simulink model "HVDC_VSC_1CPUcore_dcpl"  (Simulink 8.4)
settings: Solver=ode3  SolverMode=SingleTasking  StartTime=0.0  StopTime=70.0  FixedStep=Ts_Power  RelTol=1e-3  AbsTol=1e-2
PreLoadFcn:
  | Ts_Power=50e-6; Ts_Control=1*Ts_Power; init_cosim_IA; startup_transients_hvdc_vsc;
PostLoadFcn:
  | Ts_Power=50e-6; Ts_Control=1*Ts_Power; init_cosim_IA; startup_transients_hvdc_vsc;
InitFcn:
  | Ts_Power=50e-6; Ts_Control=1*Ts_Power; init_cosim_IA; startup_transients_hvdc_vsc;
values from neighbouring files (symbols this model uses):
  h = 5    [init_cosim_IA.m]
  intfDelay = 400.0    (= 400)    [init_cosim_IA.m]
  Ts_intf = 2*Ts_Power    [init_cosim_IA.m]
undefined symbols (not defined in the file or in its folder): CLARK, D1, Delta, dPref1_2, dPref1_2_rlimit, gcbh, level, lib_mesures, magnitude, ResistanceM, rte_drive_private_lib, rte_tsb3level_hiz_rect_cb, sps_rtmsupport, t_deblock_Pref1, t_deblock_Udref2, t_dPref1_2, t_init_AC, t_SwitchITMIdc, t_SwitchITMVdc, t_vsag_end, t_vsag_start, TSB3_hiZR
libraries: powerlib x162, powerlib_extras x71, spsVIMeasurementModel x63, rteventslib x26, op_dpl_lib x14, powerlib_meascontrol x14, rtlab x6, sps_avr x3, artemis x1
(part 1 of 11)
Description:
  | The 'Model  initialization function' defined in the
  | 
  | Model Properties automatically sets the sample time
  | 
  | Ts to 50e-6 s
settings Model: ARTEMISmethode_block_infos=$$__separator__$$HVDC_VSC_1CPUcore_dcpl/ARTEMIS Guide$$__separator__$$  Creator=Gilbert Sybille, IREQ  LastModifiedBy=maja  CovSFcnEnable=on  ExtModeTrigMode=oneshot  ExtModeArmWhenConnect=off  ExtModeAutoUpdateStatusClock=off  BufferReuse=off
settings DataIOCC: LimitDataPoints=off  SaveFormat=StructureWithTime  SaveOutput=off  DSMLogging=off  SaveTime=off  SignalLoggingName=sigsOut
settings OptimizationCC: BlockReduction=off  BooleanDataType=off  OptimizeBlockIOStorage=off  BufferReuse=off  GlobalBufferReuse=off  ExpressionFolding=off  LocalBlockOutputs=off  InitFltsAndDblsToZero=on
settings DebuggingCC: SaveWithParameterizedLinksMsg=none  CheckExecutionContextPreStartOutputMsg=on  CheckExecutionContextRuntimeOutputMsg=on  SignalResolutionControl=TryResolveAllWithWarning  SolverPrmCheckMsg=none  MultiTaskDSMMsg=warning  MultiTaskCondExecSysMsg=none  FcnCallInpInsideContextMsg=EnableAllAsWarning  UnconnectedInputMsg=none  UnconnectedOutputMsg=none  UnconnectedLineMsg=none  FrameProcessingCompatibilityMsg=error
settings HardwareCC: TargetHWDeviceType=32-bit Generic  ProdEqTarget=off
settings GRTTargetCC: TargetFcnLib=ansi_tfl_tmw.mat

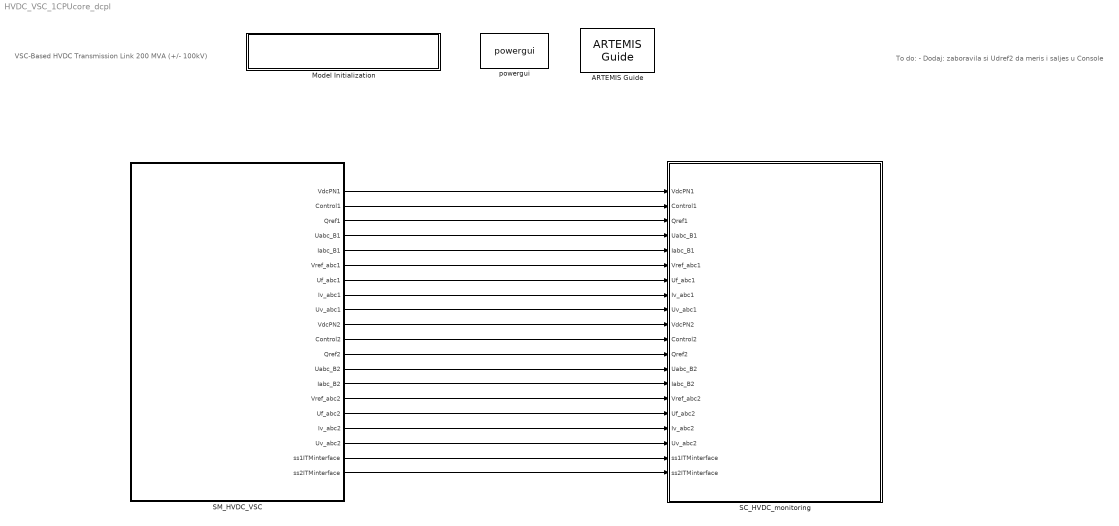
== system HVDC_VSC_1CPUcore_dcpl ==
  note: VSC-Based HVDC Transmission Link
      | 200 MVA  (+/- 100kV)
  note: To do:
      | - Dodaj: zaboravila si Udref2 da meris i saljes u Console
  ARTEMIS Guide : artemis/ARTEMIS/ARTEMIS Guide  Tag=FTSSmethode_opal_4hx0r99  Description=5.0_z1  lock=on  Ts=Ts_Power  opt=art5  dyna=off  nb_perm=4  RT_fullcomp=off  ssn=off  ssn_itvc=off  ssn_ivic=off  ssn_ext=off  ssn_solver=Trapezoidal  ssn_impulse=off  ssn_quasimpulse=off  ssn_impulse_loop=5  paraExtinctionThy=off  Thy_Impulse=on  dtc=Off  dtc_opt=normal  ao=on  simtype=off  ct_mac=off  lin_mov=off  lsp=[0.001 2]  spike_skip=Disabled  dtc_extra=1  dtc_sws=normal  dtc_pied=0.5  SPSRulesBlock=SPSRules  tre=on  ctmm=off  LF=off  dpl_type=ARTEMiS DPL  rlc_type=off  custom_type=off  para=on  ssn_ImpulseLoopBlockedStateUpdate=5  ssn_mov_iter_number=5  ssn_switch_iter_number=5
  Model Initialization : Subsystem  mask(Model Functions){InitFcnX=Ts_Power=50e-6; Ts_Control=1*Ts_Power; init_cosim_IA; startup_transients_hvdc_vsc;, prel=on, posl=on, inif=on, strf=off}
      mask prompts: InitFcnX "Initialisation"; prel "Preload Function"; posl "PostLoad Function"; inif "InitFcn"; strf "StartFcn"
      mask init:
      | currentBlock = gcb;
      | root = bdroot(currentBlock);
      | 
      | if ~strcmp(get_param(root,'BlockDiagramType'),'library')
      |     if prel==1
      |         set_param(root, 'PreLoadFcn', InitFcnX);
      |     else
      |         set_param(root, 'PreLoadFcn', '');
      |     end
      |     if inif==1
      |         set_param(root, 'InitFcn', InitFcnX);
      |     else
      |         set_param(root, 'InitFcn', '');
      |     end
      |     if strf==1
      |         set_param(root, 'StartFcn', InitFcnX);
      |     else
      |         set_param(root, 'StartFcn', '');
      |     end
      |     if posl==1
      |         set_param(root, 'PostLoadFcn', InitFcnX);
      |     else
      |         set_param(root, 'PostLoadFcn', '');
      |     end
      | end
      | 
      | pos = get_param(currentBlock, 'Position');
      | width = pos(3) - pos(1); height = pos(4) - pos(2);
      | txt = [ upper(root) '\n' '- InitFcn. . . . . '  get_param(root, 'InitFcn') ];
      settings: CopyFcn=set_param(gcb,'LinkStatus','none')
      mask Display: text(5, height*0.5, txt, 'horizontalAlignment', 'left', 'verticalAlignment', 'middle') ;
  SC_HVDC_monitoring : Subsystem
  SM_HVDC_VSC : Subsystem
  powergui : powerlib/powergui  Priority=2  SimulationMode=Discrete  SolverType=Tustin  SampleTime=Ts_Power  frequency=60  SPID=off  DisableSnubberDevices=off  DisableRonSwitches=off  DisableVfSwitches=off  SwTol=0  DisplayEquations=off  Interpol=off  methode=off  Ts=0  frequencyindice=0  Pbase=100e6  ErrMax=1e-4  Iterations=50  UnitsV=kV  UnitsW=MW  FunctionMessages=off  echomessages=on  HookPort=off  EnableUseOfTLC=off  x0status=zero  RestoreLinks=warning  ResistiveCurrentMeasurement=off  Frange=[0:2:500]  Ylog=off  Xlog=on  ShowGrid=off  save=off  variable=ZData  structure=res_fft  ZoomFFT=on  StartTime=1.5  cycles=2  DisplayStyle=1  fundamental=50  FreqAxis=off  MaxFrequency=3000  frequencyindicesteady=1  RmsSteady=1  display=off
  wires:
  SM_HVDC_VSC/1(VdcPN1) -> SC_HVDC_monitoring/1(VdcPN1)
  SM_HVDC_VSC/2(Control1) -> SC_HVDC_monitoring/2(Control1)
  SM_HVDC_VSC/3(Qref1) -> SC_HVDC_monitoring/3(Qref1)
  SM_HVDC_VSC/4(Uabc_B1) -> SC_HVDC_monitoring/4(Uabc_B1)
  SM_HVDC_VSC/5(Iabc_B1) -> SC_HVDC_monitoring/5(Iabc_B1)
  SM_HVDC_VSC/6(Vref_abc1) -> SC_HVDC_monitoring/6(Vref_abc1)
  SM_HVDC_VSC/7(Uf_abc1) -> SC_HVDC_monitoring/7(Uf_abc1)
  SM_HVDC_VSC/8(Iv_abc1) -> SC_HVDC_monitoring/8(Iv_abc1)
  SM_HVDC_VSC/9(Uv_abc1) -> SC_HVDC_monitoring/9(Uv_abc1)
  SM_HVDC_VSC/10(VdcPN2) -> SC_HVDC_monitoring/10(VdcPN2)
  SM_HVDC_VSC/11(Control2) -> SC_HVDC_monitoring/11(Control2)
  SM_HVDC_VSC/12(Qref2) -> SC_HVDC_monitoring/12(Qref2)
  SM_HVDC_VSC/13(Uabc_B2) -> SC_HVDC_monitoring/13(Uabc_B2)
  SM_HVDC_VSC/14(Iabc_B2) -> SC_HVDC_monitoring/14(Iabc_B2)
  SM_HVDC_VSC/15(Vref_abc2) -> SC_HVDC_monitoring/15(Vref_abc2)
  SM_HVDC_VSC/16(Uf_abc2) -> SC_HVDC_monitoring/16(Uf_abc2)
  SM_HVDC_VSC/17(Iv_abc2) -> SC_HVDC_monitoring/17(Iv_abc2)
  SM_HVDC_VSC/18(Uv_abc2) -> SC_HVDC_monitoring/18(Uv_abc2)
  SM_HVDC_VSC/19(ss1ITMinterface) -> SC_HVDC_monitoring/19(ss1ITMinterface)
  SM_HVDC_VSC/20(ss2ITMinterface) -> SC_HVDC_monitoring/20(ss2ITMinterface)

== system HVDC_VSC_1CPUcore_dcpl/Model Initialization ==

== system HVDC_VSC_1CPUcore_dcpl/SC_HVDC_monitoring ==
  VdcPN1 : Inport
  Control1 : Inport  Port=2
  Qref1 : Inport  Port=3
  Uabc_B1 : Inport  Port=4
  Iabc_B1 : Inport  Port=5
  Vref_abc1 : Inport  Port=6
  Uf_abc1 : Inport  Port=7
  Iv_abc1 : Inport  Port=8
  Uv_abc1 : Inport  Port=9
  VdcPN2 : Inport  Port=10
  Control2 : Inport  Port=11
  Qref2 : Inport  Port=12
  Uabc_B2 : Inport  Port=13
  Iabc_B2 : Inport  Port=14
  Vref_abc2 : Inport  Port=15
  Uf_abc2 : Inport  Port=16
  Iv_abc2 : Inport  Port=17
  Uv_abc2 : Inport  Port=18
  ss1ITMinterface : Inport  Port=19
  ss2ITMinterface : Inport  Port=20
  Bus Selector : BusSelector  OutputSignals=ss1VdcPOSf,ss1VdcNEGf,ss1VdcLINKf,ss1IdcPOSf,ss1IdcNEGf,ss1Pdcf
  Bus Selector1 : BusSelector  OutputSignals=ss2VdcPOSf,ss2VdcNEGf,ss2VdcLINKf,ss2IdcPOSf,ss2IdcNEGf,ss2Pdcf
  Data Acquisition Station 1 : Subsystem
      mask Display: disp('Open this block\nto visualize\nrecorded signals')
  Data Acquisition Station 2 : Subsystem
      mask Display: disp('Open this block\nto visualize\nrecorded signals')
  OpComm : rtlab/OpComm  nbport=9  groupe_acq=1  subsys_rate=Ts_Power  st=0  Synchronization=on  Interpolation=on  Threshold=1.0  Missed_Data=off  Sim_Time=off  Samples=off  dynSigOut=off  from_console=0  warning_done=off  writeOpCommFile=off  Offset=off
  OpComm1 : rtlab/OpComm  nbport=9  groupe_acq=2  subsys_rate=Ts_Power  st=0  Synchronization=on  Interpolation=on  Threshold=1.0  Missed_Data=off  Sim_Time=off  Samples=off  dynSigOut=off  from_console=0  warning_done=off  writeOpCommFile=off  Offset=off
  OpComm2 : rtlab/OpComm  nbport=1  groupe_acq=3  subsys_rate=Ts_Power  st=0  Synchronization=on  Interpolation=on  Threshold=1.0  Missed_Data=off  Sim_Time=off  Samples=off  dynSigOut=off  from_console=0  warning_done=off  writeOpCommFile=off  Offset=off
  OpComm3 : rtlab/OpComm  nbport=1  groupe_acq=4  subsys_rate=Ts_Power  st=0  Synchronization=on  Interpolation=on  Threshold=1.0  Missed_Data=off  Sim_Time=off  Samples=off  dynSigOut=off  from_console=0  warning_done=off  writeOpCommFile=off  Offset=off
  Subsystem : Subsystem
  wires:
  VdcPN1/1 -> OpComm/1
  Control1/1 -> OpComm/2
  Qref1/1 -> OpComm/3
  Uabc_B1/1 -> OpComm/4
  Iabc_B1/1 -> OpComm/5
  Vref_abc1/1 -> OpComm/6
  Uf_abc1/1 -> OpComm/7
  Iv_abc1/1 -> OpComm/8
  Uv_abc1/1 -> OpComm/9
  OpComm/1 -> Data Acquisition Station 1/1(VdcPN1)
  OpComm/2 -> Data Acquisition Station 1/2(Control1)
  OpComm/3 -> Data Acquisition Station 1/3(Qref1)
  OpComm/4 -> Data Acquisition Station 1/4(Uabc_B1)
  OpComm/5 -> Data Acquisition Station 1/5(Iabc_B1)
  OpComm/6 -> Data Acquisition Station 1/6(Vref_abc1)
  OpComm/7 -> Data Acquisition Station 1/7(Uf_abc1)
  OpComm/8 -> Data Acquisition Station 1/8(Iv_abc1)
  OpComm/9 -> Data Acquisition Station 1/9(Uv_abc1)
  VdcPN2/1 -> OpComm1/1
  Control2/1 -> OpComm1/2
  Qref2/1 -> OpComm1/3
  Uabc_B2/1 -> OpComm1/4
  Iabc_B2/1 -> OpComm1/5
  Vref_abc2/1 -> OpComm1/6
  Uf_abc2/1 -> OpComm1/7
  Iv_abc2/1 -> OpComm1/8
  Uv_abc2/1 -> OpComm1/9
  OpComm1/1 -> Data Acquisition Station 2/1(VdcPN2)
  OpComm1/2 -> Data Acquisition Station 2/2(Control2)
  OpComm1/3 -> Data Acquisition Station 2/3(Qref2)
  OpComm1/4 -> Data Acquisition Station 2/4(Uabc_B2)
  OpComm1/5 -> Data Acquisition Station 2/5(Iabc_B2)
  OpComm1/6 -> Data Acquisition Station 2/6(Vref_abc2)
  OpComm1/7 -> Data Acquisition Station 2/7(Uf_abc2)
  OpComm1/8 -> Data Acquisition Station 2/8(Iv_abc2)
  OpComm1/9 -> Data Acquisition Station 2/9(Uv_abc2)
  ss1ITMinterface/1 -> OpComm2/1
  OpComm2/1 -> Bus Selector/1
  ss2ITMinterface/1 -> OpComm3/1
  OpComm3/1 -> Bus Selector1/1
  Bus Selector/1 -> Subsystem/1(In1)  "<ss1VdcPOSf>"
  Bus Selector/2 -> Subsystem/2(In2)  "<ss1VdcNEGf>"
  Bus Selector/3 -> Subsystem/3(In3)  "<ss1VdcLINKf>"
  Bus Selector/4 -> Subsystem/4(In4)  "<ss1IdcPOSf>"
  Bus Selector/5 -> Subsystem/5(In5)  "<ss1IdcNEGf>"
  Bus Selector/6 -> Subsystem/6(In6)  "<ss1Pdcf>"
  Bus Selector1/1 -> Subsystem/7(In7)  "<ss2VdcPOSf>"
  Bus Selector1/2 -> Subsystem/8(In8)  "<ss2VdcNEGf>"
  Bus Selector1/3 -> Subsystem/9(In9)  "<ss2VdcLINKf>"
  Bus Selector1/4 -> Subsystem/10(In10)  "<ss2IdcPOSf>"
  Bus Selector1/5 -> Subsystem/11(In11)  "<ss2IdcNEGf>"
  Bus Selector1/6 -> Subsystem/12(In12)  "<ss2Pdcf>"

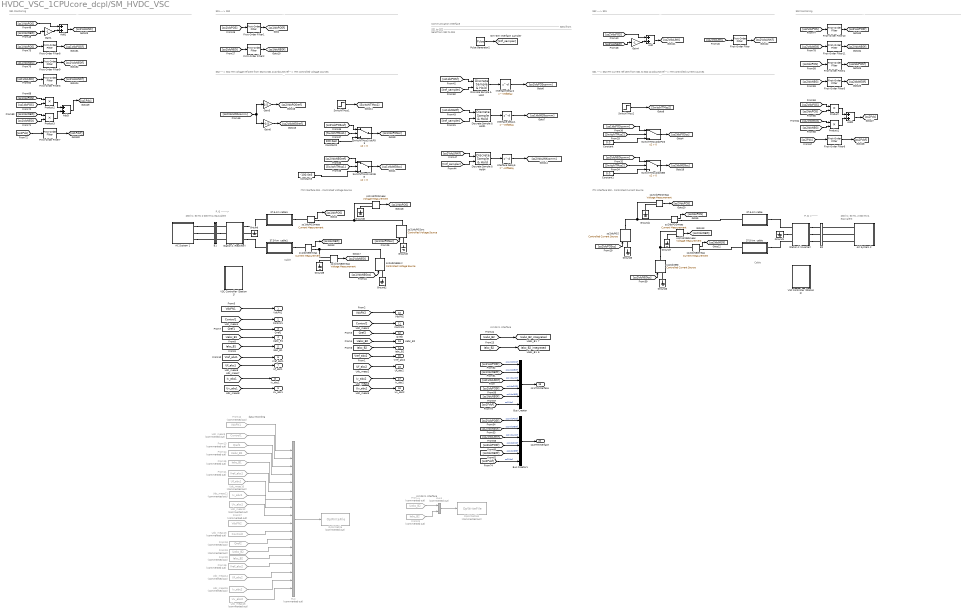
== system HVDC_VSC_1CPUcore_dcpl/SM_HVDC_VSC ==
  note: sim2sim interface
  note: 230 kV, 50 Hz
      |  2 000 MVA equivalent
  note: P, Q
      | <------
  note: P, Q
      | ------>
  note: Cable
  note: 230 kV, 50 Hz,
      | 2 000 MVA equivalent
  note: sim2sim interface
  note: data recording
  note: Cable
  note: SS2 ---> SS1
      | ITM voltage ref sent from SS2 to SS1
      | ss2VdcLINKref
      | --> ITM controlled voltage sources
      | ------------------------------------------------------------------------------------------------------------------------------------------------------------------------------------
  note: Communication Interface
      |
      | --------------------------------------------------------------------------------------------------------------------------------
      | Send from SS1 to SS2
      |
      | --------------------------------------------------------------------------------------------------------------------------------
      | Send from SS2 to SS1
  note: SS1 ---> SS2
      | ------------------------------------------------------------------------------------------------------------------------------------------------------------------------------------
  note: SS2 ---> SS1
      | ------------------------------------------------------------------------------------------------------------------------------------------------------------------------------------
  note: SS1 ---> SS2
      | ITM current ref sent from SS1 to SS2
      | ss1IdcLINKref
      | --> ITM controlled current sources
      | ------------------------------------------------------------------------------------------------------------------------------------------------------------------------------------
  note: ITM Interface SS1 - Controlled Voltage Source
  note: ITM Interface SS2 - Controlled Current Source
  note: SS1 Monitoring
      | ------------------------------------------------------------------------------------------------------------------------------------------------------------------------------------
  note: SS2 Monitoring
      | ------------------------------------------------------------------------------------------------------------------------------------------------------------------------------------
  37.5-km  cable : Subsystem  mask(Artemis Distributed Parameters Line){SimulationMode=ARTEMIS model, Phases=1, Frequency=60, Resistance=1.3900e-002, Inductance=1.5900e-004, Capacitance=2.3100e-007, Length=37.5, Measurements=None}
      mask prompts: SimulationMode "Simulation Mode"; Phases "Number of phases N"; Frequency "Frequency used for R L C specification (Hz)"; Resistance "Resistance per unit length (Ohms/km)   [N*N matrix] or [R1 R0 R0m]"; Inductance "Inductance per unit length (H/km) [N*N matrix ] or [L1 L0 L0m]"; Capacitance "Capacitance per unit length (F/km) [N*N matrix] or [C1 C0 C0m]"; Length "Line length (km)"
      mask help:
      | Implements a N-phases distributed parameter line model. The R,L, and C line parameters are specified by [NxN] matrices.
      |
      | To model a two-, three-, or a six-phase symetrical line you can either specify complete [NxN] matrices or simply enter sequence parameters vectors: the  positive and zero sequence parameters for a two-phase or  three-phase transposed  line, plus the mutual zero-sequence for a  six-phase transposed  line  (2 coupled 3-phase lines).
      mask init:
      | % Get current block
      | currentBlock = gcb;
      | 
      | % Get electric variables
      | [Zm,R,v,Ti,to,Rt4,h,Zimp,Zmat,Yphase,ResistanceM] = op_distributedparametersline_cb(gcb,'variable_mask_maskinitialization', Phases, Frequency, Resistance, Inductance, Capacitance, Length);
      | 
      | % Set block contents
      | op_distributedparametersline_cb(currentBlock,'maskinitialization');
      mask Help: eval('fts2help(''distributedparametersline'');');
      mask TypeOptions SimulationMode: SimPowerSystems model | ARTEMIS model
      mask TypeOptions Phases: 1 | 2 | 3 | 4 | 5 | 6
      mask TypeOptions Measurements: None
      mask Display:
      | patch([0 0.5 0.7 0],[1 1 0 0],[0.7 0.75 0.9]);
      | patch([1 0.53 0.73 1],[1 1 0 0],[1 0.8 0.7]);
      | plot([0 0 1 1 0],[0 1 1 0 0]);
      | plot([0 0.2 0.2 0.8 0.8 1 0.8 0.8 0.2 0.2 NaN 0 NaN 1],[0.5 0.5 0.625 0.625 0.5 0.5 0.5 0.375 0.375 0.5 NaN 0 NaN 1])
      | disp('DPL')
  37.5-km  cable1 : Subsystem  mask(Artemis Distributed Parameters Line){SimulationMode=ARTEMIS model, Phases=1, Frequency=60, Resistance=1.3900e-002, Inductance=1.5900e-004, Capacitance=2.3100e-007, Length=37.5, Measurements=None}
      mask prompts: SimulationMode "Simulation Mode"; Phases "Number of phases N"; Frequency "Frequency used for R L C specification (Hz)"; Resistance "Resistance per unit length (Ohms/km)   [N*N matrix] or [R1 R0 R0m]"; Inductance "Inductance per unit length (H/km) [N*N matrix ] or [L1 L0 L0m]"; Capacitance "Capacitance per unit length (F/km) [N*N matrix] or [C1 C0 C0m]"; Length "Line length (km)"
      mask help:
      | Implements a N-phases distributed parameter line model. The R,L, and C line parameters are specified by [NxN] matrices.
      |
      | To model a two-, three-, or a six-phase symetrical line you can either specify complete [NxN] matrices or simply enter sequence parameters vectors: the  positive and zero sequence parameters for a two-phase or  three-phase transposed  line, plus the mutual zero-sequence for a  six-phase transposed  line  (2 coupled 3-phase lines).
      mask init: same as HVDC_VSC_1CPUcore_dcpl/SM_HVDC_VSC/37.5-km  cable
      mask Help: eval('fts2help(''distributedparametersline'');');
      mask TypeOptions SimulationMode: SimPowerSystems model | ARTEMIS model
      mask TypeOptions Phases: 1 | 2 | 3 | 4 | 5 | 6
      mask TypeOptions Measurements: None
      mask Display:
      | patch([0 0.5 0.7 0],[1 1 0 0],[0.7 0.75 0.9]);
      | patch([1 0.53 0.73 1],[1 1 0 0],[1 0.8 0.7]);
      | plot([0 0 1 1 0],[0 1 1 0 0]);
      | plot([0 0.2 0.2 0.8 0.8 1 0.8 0.8 0.2 0.2 NaN 0 NaN 1],[0.5 0.5 0.625 0.625 0.5 0.5 0.5 0.375 0.375 0.5 NaN 0 NaN 1])
      | disp('DPL')
  37.5-km cable : Subsystem  mask(Artemis Distributed Parameters Line){SimulationMode=ARTEMIS model, Phases=1, Frequency=60, Resistance=1.3900e-002, Inductance=1.5900e-004, Capacitance=2.3100e-007, Length=37.5, Measurements=None}
      mask prompts: SimulationMode "Simulation Mode"; Phases "Number of phases N"; Frequency "Frequency used for R L C specification (Hz)"; Resistance "Resistance per unit length (Ohms/km)   [N*N matrix] or [R1 R0 R0m]"; Inductance "Inductance per unit length (H/km) [N*N matrix ] or [L1 L0 L0m]"; Capacitance "Capacitance per unit length (F/km) [N*N matrix] or [C1 C0 C0m]"; Length "Line length (km)"
      mask help:
      | Implements a N-phases distributed parameter line model. The R,L, and C line parameters are specified by [NxN] matrices.
      |
      | To model a two-, three-, or a six-phase symetrical line you can either specify complete [NxN] matrices or simply enter sequence parameters vectors: the  positive and zero sequence parameters for a two-phase or  three-phase transposed  line, plus the mutual zero-sequence for a  six-phase transposed  line  (2 coupled 3-phase lines).
      mask init: same as HVDC_VSC_1CPUcore_dcpl/SM_HVDC_VSC/37.5-km  cable
      mask Help: eval('fts2help(''distributedparametersline'');');
      mask TypeOptions SimulationMode: SimPowerSystems model | ARTEMIS model
      mask TypeOptions Phases: 1 | 2 | 3 | 4 | 5 | 6
      mask TypeOptions Measurements: None
      mask Display:
      | patch([0 0.5 0.7 0],[1 1 0 0],[0.7 0.75 0.9]);
      | patch([1 0.53 0.73 1],[1 1 0 0],[1 0.8 0.7]);
      | plot([0 0 1 1 0],[0 1 1 0 0]);
      | plot([0 0.2 0.2 0.8 0.8 1 0.8 0.8 0.2 0.2 NaN 0 NaN 1],[0.5 0.5 0.625 0.625 0.5 0.5 0.5 0.375 0.375 0.5 NaN 0 NaN 1])
      | disp('DPL')
  37.5-km cable1 : Subsystem  mask(Artemis Distributed Parameters Line){SimulationMode=ARTEMIS model, Phases=1, Frequency=60, Resistance=1.3900e-002, Inductance=1.5900e-004, Capacitance=2.3100e-007, Length=37.5, Measurements=None}
      mask prompts: SimulationMode "Simulation Mode"; Phases "Number of phases N"; Frequency "Frequency used for R L C specification (Hz)"; Resistance "Resistance per unit length (Ohms/km)   [N*N matrix] or [R1 R0 R0m]"; Inductance "Inductance per unit length (H/km) [N*N matrix ] or [L1 L0 L0m]"; Capacitance "Capacitance per unit length (F/km) [N*N matrix] or [C1 C0 C0m]"; Length "Line length (km)"
      mask help:
      | Implements a N-phases distributed parameter line model. The R,L, and C line parameters are specified by [NxN] matrices.
      |
      | To model a two-, three-, or a six-phase symetrical line you can either specify complete [NxN] matrices or simply enter sequence parameters vectors: the  positive and zero sequence parameters for a two-phase or  three-phase transposed  line, plus the mutual zero-sequence for a  six-phase transposed  line  (2 coupled 3-phase lines).
      mask init: same as HVDC_VSC_1CPUcore_dcpl/SM_HVDC_VSC/37.5-km  cable
      mask Help: eval('fts2help(''distributedparametersline'');');
      mask TypeOptions SimulationMode: SimPowerSystems model | ARTEMIS model
      mask TypeOptions Phases: 1 | 2 | 3 | 4 | 5 | 6
      mask TypeOptions Measurements: None
      mask Display:
      | patch([0 0.5 0.7 0],[1 1 0 0],[0.7 0.75 0.9]);
      | patch([1 0.53 0.73 1],[1 1 0 0],[1 0.8 0.7]);
      | plot([0 0 1 1 0],[0 1 1 0 0]);
      | plot([0 0.2 0.2 0.8 0.8 1 0.8 0.8 0.2 0.2 NaN 0 NaN 1],[0.5 0.5 0.625 0.625 0.5 0.5 0.5 0.375 0.375 0.5 NaN 0 NaN 1])
      | disp('DPL')
  AC System 1 : Subsystem
  AC System 2 : Subsystem
  Add{,1..3} (4 alike) : Sum
  B1 : Subsystem  DialogController=POWERSYS.PowerSysDialog  LoadFcn=sps_rtmsupport('LoadFcn',gcbh);  StartFcn=sps_rtmsupport('StartFcn',gcbh);  StopFcn=sps_rtmsupport('StopFcn',gcbh);  mask(Three-Phase VI Measurement){VoltageMeasurement=phase-to-ground, SetLabelV=on, LabelV=Uabc_B1, Vpu=on, VpuLL=off, CurrentMeasurement=yes, SetLabelI=on, LabelI=Iabc_B1, Ipu=on, Pbase=200e6, Vbase=230e3, OutputType=Magnitude, PhasorSimulation=off, PSBequivalent=0}
      mask prompts: VoltageMeasurement "Voltage measurement"; SetLabelV "Use a label"; LabelV "Signal label  (use a From block to collect this signal)"; Vpu "Voltages in pu,  based on peak value of nominal phase-to-ground voltage"; VpuLL "Voltages in pu,  based on peak value of nominal phase-to-phase  voltage"; CurrentMeasurement "Current measurement"; SetLabelI "Use a label"; LabelI "Signal label  (use a From block to collect this signal)"; Ipu "Currents in pu"; Pbase "Base power ( VA 3 phase)"; Vbase "Nominal voltage used for pu measurement (Vrms phase-phase) :"; OutputType "Output signals in:"; PhasorSimulation "Phasor simulation (internal use)"; PSBequivalent "Equivalent circuit (internal use)"
      mask help:
      | Ideal three-phase voltage and current measurements.
      |
      | The block can output the voltages and currents in per unit values or in volts and amperes.
      mask init:
      | block = gcb;
      | Kv=1;
      | Ki=1;
      | [Kv,Ki] = powericon('ThreePhaseVIMeasurementParam',block,Vpu,VpuLL,Ipu,Vbase,Pbase,PhasorSimulation,OutputType);
      | powericon('ThreePhaseVIMeasurementCback',block);
      | power_initmask();
      settings: CopyFcn=sps_rtmsupport('CopyFcn',gcbh); powericon('ThreePhaseVIMeasurementCopy',gcb)  DeleteFcn=sps_rtmsupport('DeleteFcn',gcbh);  UndoDeleteFcn=sps_rtmsupport('UndoDeleteFcn',gcbh);  ModelCloseFcn=sps_rtmsupport('ModelCloseFcn',gcbh);  PreSaveFcn="sps_rtmsupport('PreSaveFcn',gcbh);  set_param(gcb,'LinkStatus','restore')"  PostSaveFcn=sps_rtmsupport('PostSaveFcn',gcbh);  NameChangeFcn=sps_rtmsupport('NameChangeFcn',gcbh);  PreCopyFcn=sps_rtmsupport('PreCopyFcn',gcbh);  OpenFcn=sps_rtmsupport('OpenFcn',gcbh, [1 2 4 5 6 7 9 -12 13]);  CloseFcn=sps_rtmsupport('CloseFcn',gcbh);  PreDeleteFcn=sps_rtmsupport('PreDeleteFcn',gcbh);
      mask Help: helpview(psbhelp)
      mask TypeOptions VoltageMeasurement: no | phase-to-ground | phase-to-phase
      mask Callback VoltageMeasurement: powericon('ThreePhaseVIMeasurementCback',gcb,'Vselector');
      mask Callback SetLabelV: powericon('ThreePhaseVIMeasurementCback',gcb,'');
      mask Callback Vpu: powericon('ThreePhaseVIMeasurementCback',gcb,'Vpu');
      mask Callback VpuLL: powericon('ThreePhaseVIMeasurementCback',gcb,'VpuLL');
      mask TypeOptions CurrentMeasurement: no | yes
      mask Callback CurrentMeasurement: powericon('ThreePhaseVIMeasurementCback',gcb,'');
      mask Callback SetLabelI: powericon('ThreePhaseVIMeasurementCback',gcb,'');
      mask Callback LabelI: powericon('ThreePhaseVIMeasurementCback',gcb,'');
      mask Callback Ipu: powericon('ThreePhaseVIMeasurementCback',gcb,'');
      mask TypeOptions OutputType: Complex | Real-Imag | Magnitude-Angle | Magnitude
  B2 : Subsystem  DialogController=POWERSYS.PowerSysDialog  LoadFcn=sps_rtmsupport('LoadFcn',gcbh);  StartFcn=sps_rtmsupport('StartFcn',gcbh);  StopFcn=sps_rtmsupport('StopFcn',gcbh);  mask(Three-Phase VI Measurement){VoltageMeasurement=phase-to-ground, SetLabelV=on, LabelV=Uabc_B2, Vpu=on, VpuLL=off, CurrentMeasurement=yes, SetLabelI=on, LabelI=Iabc_B2, Ipu=on, Pbase=200e6, Vbase=230e3, OutputType=Magnitude, PhasorSimulation=off, PSBequivalent=0}
      mask prompts: VoltageMeasurement "Voltage measurement"; SetLabelV "Use a label"; LabelV "Signal label  (use a From block to collect this signal)"; Vpu "Voltages in pu,  based on peak value of nominal phase-to-ground voltage"; VpuLL "Voltages in pu,  based on peak value of nominal phase-to-phase  voltage"; CurrentMeasurement "Current measurement"; SetLabelI "Use a label"; LabelI "Signal label  (use a From block to collect this signal)"; Ipu "Currents in pu"; Pbase "Base power ( VA 3 phase)"; Vbase "Nominal voltage used for pu measurement (Vrms phase-phase) :"; OutputType "Output signals in:"; PhasorSimulation "Phasor simulation (internal use)"; PSBequivalent "Equivalent circuit (internal use)"
      mask help:
      | Ideal three-phase voltage and current measurements.
      |
      | The block can output the voltages and currents in per unit values or in volts and amperes.
      mask init: same as HVDC_VSC_1CPUcore_dcpl/SM_HVDC_VSC/B1
      settings: CopyFcn=sps_rtmsupport('CopyFcn',gcbh); powericon('ThreePhaseVIMeasurementCopy',gcb)  DeleteFcn=sps_rtmsupport('DeleteFcn',gcbh);  UndoDeleteFcn=sps_rtmsupport('UndoDeleteFcn',gcbh);  ModelCloseFcn=sps_rtmsupport('ModelCloseFcn',gcbh);  PreSaveFcn="sps_rtmsupport('PreSaveFcn',gcbh);  set_param(gcb,'LinkStatus','restore')"  PostSaveFcn=sps_rtmsupport('PostSaveFcn',gcbh);  NameChangeFcn=sps_rtmsupport('NameChangeFcn',gcbh);  PreCopyFcn=sps_rtmsupport('PreCopyFcn',gcbh);  OpenFcn=sps_rtmsupport('OpenFcn',gcbh, [1 2 4 5 6 7 9 -12 13]);  CloseFcn=sps_rtmsupport('CloseFcn',gcbh);  PreDeleteFcn=sps_rtmsupport('PreDeleteFcn',gcbh);
      mask Help: helpview(psbhelp)
      mask TypeOptions VoltageMeasurement: no | phase-to-ground | phase-to-phase
      mask Callback VoltageMeasurement: powericon('ThreePhaseVIMeasurementCback',gcb,'Vselector');
      mask Callback SetLabelV: powericon('ThreePhaseVIMeasurementCback',gcb,'');
      mask Callback Vpu: powericon('ThreePhaseVIMeasurementCback',gcb,'Vpu');
      mask Callback VpuLL: powericon('ThreePhaseVIMeasurementCback',gcb,'VpuLL');
      mask TypeOptions CurrentMeasurement: no | yes
      mask Callback CurrentMeasurement: powericon('ThreePhaseVIMeasurementCback',gcb,'');
      mask Callback SetLabelI: powericon('ThreePhaseVIMeasurementCback',gcb,'');
      mask Callback LabelI: powericon('ThreePhaseVIMeasurementCback',gcb,'');
      mask Callback Ipu: powericon('ThreePhaseVIMeasurementCback',gcb,'');
      mask TypeOptions OutputType: Complex | Real-Imag | Magnitude-Angle | Magnitude
  Bus Creator : BusCreator  Inputs=6
  Bus Creator1 : BusCreator  Inputs=6
  Constant : Constant  Value=0.0
  Constant1 : Constant  Value=0.0
  Constant2 : Constant  Value=100.0e3
  Constant3 : Constant  Value=-100.0e3
  Discrete Sample & Hold : powerlib_extras/Discrete  Control Blocks/Discrete Sample & Hold  ic=0  Ts=Ts_intf
  Discrete Sample & Hold1 : powerlib_extras/Discrete  Control Blocks/Discrete Sample & Hold  ic=0  Ts=Ts_intf
  Discrete Sample & Hold4 : powerlib_extras/Discrete  Control Blocks/Discrete Sample & Hold  ic=0  Ts=Ts_intf
  First-Order Filter{,1..11} (12 alike) : powerlib_meascontrol/Filters/First-Order Filter  FilterType=Lowpass  Tc=0.05  Ts=Ts_Power  Initialize=on  Vac_Init=[0, 0, 0]  Vdc_Init=0  PlotResponse=off  FreqRange="[0,  200,  1]"
  From11 : From  Commented=on  GotoTag=Vref_abc1  TagVisibility=global
      settings: CloseFcn=tagdialog Close
  From12 : From  Commented=on  GotoTag=VdcPN1  TagVisibility=global
      settings: CloseFcn=tagdialog Close
  From13 : From  Commented=on  GotoTag=Qref1  TagVisibility=global
      settings: CloseFcn=tagdialog Close
  From14 : From  Commented=on  GotoTag=Uabc_B1  TagVisibility=global
      settings: CloseFcn=tagdialog Close
  From15 : From  Commented=on  GotoTag=Iabc_B1  TagVisibility=global
      settings: CloseFcn=tagdialog Close
  From16 : From  Commented=on  GotoTag=Vref_abc2  TagVisibility=global
      settings: CloseFcn=tagdialog Close
  From17 : From  Commented=on  GotoTag=VdcPN2  TagVisibility=global
      settings: CloseFcn=tagdialog Close
  From18 : From  Commented=on  GotoTag=Qref2  TagVisibility=global
      settings: CloseFcn=tagdialog Close
  From19 : From  Commented=on  GotoTag=Uabc_B2  TagVisibility=global
      settings: CloseFcn=tagdialog Close
  From20 : From  Commented=on  GotoTag=Iabc_B2  TagVisibility=global
      settings: CloseFcn=tagdialog Close
  From21 : From  Commented=on  GotoTag=Iabc_B2  TagVisibility=global
      settings: CloseFcn=tagdialog Close
  From22 : From  Commented=on  GotoTag=Uabc_B2  TagVisibility=global
      settings: CloseFcn=tagdialog Close
  Gain1 : Gain  Gain=-1
  Gain4 : Gain  Gain=-1
  Gain5 : Gain  Gain=0.5
  Gain6 : Gain  Gain=-0.5
  Ground{,1..9} (10 alike) : powerlib/Elements/Ground  LConnTagsString=a
  Interface Delay1 : Delay  DelayLength=intfDelay  InputProcessing=Inherited
  Interface Delay2 : Delay  DelayLength=intfDelay  InputProcessing=Inherited
  Interface Delay5 : Delay  DelayLength=intfDelay  InputProcessing=Inherited
  Mux : Mux  Commented=on  Inputs=18
  Mux1 : Mux  Commented=on  Inputs=2
  OpWriteFile : rtlab/DataLogging/OpWriteFile  Commented=on  Static_File=on  varname=opvar_HVDC_integrated  Filename=HVDC_integrated.mat  rtpath='./'  nrtpath='.\'  Acq_Group=26  file_size=75000000  write_offline=off  Sim_Mode=off  Nb_Samples=5000  Buffer_size=4000000
      settings: Decimation=3
  OpWriteFile1 : rtlab/DataLogging/OpWriteFile  Commented=on  Static_File=on  varname=opvar_HVDC_integrated_intf  Filename=HVDC_integrated_intf.mat  rtpath='./'  nrtpath='.\'  Acq_Group=27  file_size=75000000  write_offline=off  Sim_Mode=off  Nb_Samples=5000  Buffer_size=4000000
      settings: Decimation=3
  Product{,1..3} (4 alike) : Product
  Pulse Generator2 : DiscretePulseGenerator  Period=h  SampleTime=Ts_intf
  Station 1 (Rectifier) : Subsystem
  Station 2 (Inverter) : Subsystem
  SwitchITMss1 : Step  Time=t_SwitchITMVdc  SampleTime=Ts_Control
  SwitchITMss1VdcNEG : Switch  Criteria=u2 > Threshold
  SwitchITMss1VdcPOS : Switch  Criteria=u2 > Threshold
  SwitchITMss2 : Step  Time=t_SwitchITMIdc  SampleTime=Ts_Control
  SwitchITMss2IdcNEG : Switch  Criteria=u2 > Threshold
  SwitchITMss2IdcPOS : Switch  Criteria=u2 > Threshold
  Udc_meas10 : From  Commented=on  GotoTag=Uf_abc1  TagVisibility=global
      settings: CloseFcn=tagdialog Close
  Udc_meas11 : From  Commented=on  GotoTag=Iv_abc1  TagVisibility=global
      settings: CloseFcn=tagdialog Close
  Udc_meas12 : From  Commented=on  GotoTag=Uv_abc1  TagVisibility=global
      settings: CloseFcn=tagdialog Close
  Udc_meas13 : From  Commented=on  GotoTag=Control2  TagVisibility=global
      settings: CloseFcn=tagdialog Close
  Udc_meas14 : From  Commented=on  GotoTag=Uf_abc2  TagVisibility=global
      settings: CloseFcn=tagdialog Close
  Udc_meas15 : From  Commented=on  GotoTag=Iv_abc2  TagVisibility=global
      settings: CloseFcn=tagdialog Close
  Udc_meas16 : From  Commented=on  GotoTag=Uv_abc2  TagVisibility=global
      settings: CloseFcn=tagdialog Close
  Udc_meas9 : From  Commented=on  GotoTag=Control1  TagVisibility=global
      settings: CloseFcn=tagdialog Close
  VSC Controller (Station 1) : Subsystem
  VSC Controller (Station 2) : Subsystem
  ss1IdcNEGmeas : powerlib/Measurements/Current Measurement  PhasorSimulation=off  OutputType=Complex  PSBequivalent=0
  ss1IdcPOSmeas : powerlib/Measurements/Current Measurement  PhasorSimulation=off  OutputType=Complex  PSBequivalent=0
  ss1VdcNEGmeas : powerlib/Measurements/Voltage Measurement  PhasorSimulation=off  OutputType=Complex  PSBequivalent=0
  ss1VdcPOSmeas : powerlib/Measurements/Voltage Measurement  PhasorSimulation=off  OutputType=Complex  PSBequivalent=0
  ss2IdcNEG : powerlib/Electrical Sources/Controlled Current Source  Initialize=on  Source_Type=DC  Amplitude=0.0  Phase=0  Frequency=0  Measurements=None
  ss2IdcNEGmeas : powerlib/Measurements/Current Measurement  PhasorSimulation=off  OutputType=Complex  PSBequivalent=0
  ss2IdcPOS : powerlib/Electrical Sources/Controlled Current Source  Initialize=on  Source_Type=DC  Amplitude=0.0  Phase=0  Frequency=0  Measurements=None
  ss2IdcPOSmeas : powerlib/Measurements/Current Measurement  PhasorSimulation=off  OutputType=Complex  PSBequivalent=0
  ss2UdcNEGsrc : powerlib/Electrical Sources/Controlled Voltage Source  Initialize=on  Source_Type=DC  Amplitude=-100.0e3  Phase=0  Frequency=0  Measurements=None
  ss2UdcPOSsrc : powerlib/Electrical Sources/Controlled Voltage Source  Initialize=on  Source_Type=DC  Amplitude=100.0e3  Phase=0  Frequency=0  Measurements=None
  ss2VdcNEGmeas : powerlib/Measurements/Voltage Measurement  PhasorSimulation=off  OutputType=Complex  PSBequivalent=0
  ss2VdcPOSmeas : powerlib/Measurements/Voltage Measurement  PhasorSimulation=off  OutputType=Complex  PSBequivalent=0
  VdcPN1 : Outport
  Control1 : Outport  Port=2
  Qref1 : Outport  Port=3
  Uabc_B1 : Outport  Port=4
  Iabc_B1 : Outport  Port=5
  Vref_abc1 : Outport  Port=6
  Uf_abc1 : Outport  Port=7
  Iv_abc1 : Outport  Port=8
  Uv_abc1 : Outport  Port=9
  VdcPN2 : Outport  Port=10
  Control2 : Outport  Port=11
  Qref2 : Outport  Port=12
  Uabc_B2 : Outport  Port=13
  Iabc_B2 : Outport  Port=14
  Vref_abc2 : Outport  Port=15
  Uf_abc2 : Outport  Port=16
  Iv_abc2 : Outport  Port=17
  Uv_abc2 : Outport  Port=18
  ss1ITMinterface : Outport  Port=19
  ss2ITMinterface : Outport  Port=20
  tag scope: Iabc_B2_integrated=global, Uabc_B2_integrated=global
  wires:
  [Iabc_B2] -> [Iabc_B2_integrated]
  [Uabc_B2] -> [Uabc_B2_integrated]
  [VdcPN1] -> VdcPN1/1
  [Uv_abc2] -> Uv_abc2/1
  [Iv_abc2] -> Iv_abc2/1
  [Uf_abc2] -> Uf_abc2/1
  [Vref_abc2] -> Vref_abc2/1
  [Iabc_B2] -> Iabc_B2/1
  [Uabc_B2] -> Uabc_B2/1
  [Qref2] -> Qref2/1
  [Control2] -> Control2/1
  [VdcPN2] -> VdcPN2/1
  [Uv_abc1] -> Uv_abc1/1
  [Iv_abc1] -> Iv_abc1/1
  [Uf_abc1] -> Uf_abc1/1
  [Vref_abc1] -> Vref_abc1/1
  [Iabc_B1] -> Iabc_B1/1
  [Uabc_B1] -> Uabc_B1/1
  [Qref1] -> Qref1/1
  [Control1] -> Control1/1
  From12/1 -> Mux/1
  Udc_meas9/1 -> Mux/2
  From13/1 -> Mux/3
  From14/1 -> Mux/4
  From15/1 -> Mux/5
  From11/1 -> Mux/6
  Udc_meas10/1 -> Mux/7
  Udc_meas11/1 -> Mux/8
  Udc_meas12/1 -> Mux/9
  From17/1 -> Mux/10
  Udc_meas13/1 -> Mux/11
  From18/1 -> Mux/12
  From19/1 -> Mux/13
  From20/1 -> Mux/14
  From16/1 -> Mux/15
  Udc_meas14/1 -> Mux/16
  Udc_meas15/1 -> Mux/17
  Udc_meas16/1 -> Mux/18
  Mux/1 -> OpWriteFile/1
  From22/1 -> Mux1/1
  From21/1 -> Mux1/2
  Mux1/1 -> OpWriteFile1/1
  ss2VdcNEGmeas/1 -> [ss2VdcNEG]
  ss2VdcPOSmeas/1 -> [ss2VdcPOS]
  ss1IdcPOSmeas/1 -> [ss1IdcPOS]
  ss1IdcNEGmeas/1 -> [ss1IdcNEG]
  [ss2IdcNEGcc] -> ss2IdcNEG/1
  [ss2IdcPOScc] -> ss2IdcPOS/1
  Discrete Sample & Hold/1 -> Interface Delay2/1
  Interface Delay2/1 -> [ss1IdcPOScomm]
  Pulse Generator2/1 -> [Intf_sampler]
  Interface Delay1/1 -> [ss1IdcNEGcomm]
  [Intf_sampler] -> Discrete Sample & Hold1/2
  Discrete Sample & Hold1/1 -> Interface Delay1/1
  SwitchITMss2IdcPOS/1 -> [ss2IdcPOScc]
  Constant/1 -> SwitchITMss2IdcPOS/3
  [SwitchITMss2] -> SwitchITMss2IdcPOS/2
  Constant1/1 -> SwitchITMss2IdcNEG/3
  [SwitchITMss2] -> SwitchITMss2IdcNEG/2
  Constant3/1 -> SwitchITMss1VdcNEG/3
  [ss2VdcNEGref] -> SwitchITMss1VdcNEG/1
  Constant2/1 -> SwitchITMss1VdcPOS/3
  [ss2VdcPOSref] -> SwitchITMss1VdcPOS/1
  SwitchITMss1VdcPOS/1 -> [ss1VdcPOScc]
  [SwitchITMss1] -> SwitchITMss1VdcPOS/2
  [SwitchITMss1] -> SwitchITMss1VdcNEG/2
  [ss1VdcPOScc] -> ss2UdcPOSsrc/1
  [ss1VdcNEGcc] -> ss2UdcNEGsrc/1
  SwitchITMss1/1 -> [SwitchITMss1]
  SwitchITMss2/1 -> [SwitchITMss2]
  ss2IdcPOSmeas/1 -> [ss2IdcPOS]
  ss1VdcPOSmeas/1 -> [ss1VdcPOS]
  ss1VdcNEGmeas/1 -> [ss1VdcNEG]
  Discrete Sample & Hold4/1 -> Interface Delay5/1
  Interface Delay5/1 -> [ss2VdcLINKcomm]
  [ss2VdcNEG] -> Gain4/1
  [ss2VdcPOS] -> Add/1
  Gain4/1 -> Add/2
  [ss2VdcLINKcomm] -> Gain5/1, Gain6/1
  Gain6/1 -> [ss2VdcNEGref]
  Gain5/1 -> [ss2VdcPOSref]
  [ss1IdcPOScomm] -> SwitchITMss2IdcPOS/1
  [ss1IdcNEGcomm] -> SwitchITMss2IdcNEG/1
  ss2IdcNEGmeas/1 -> [ss2IdcNEG]
  [ss1IdcPOS] -> First-Order Filter1/1
  [ss1IdcNEG] -> First-Order Filter2/1
  SwitchITMss2IdcNEG/1 -> [ss2IdcNEGcc]
  SwitchITMss1VdcNEG/1 -> [ss1VdcNEGcc]
  First-Order Filter1/1 -> [ss1IdcPOSf]
  First-Order Filter2/1 -> [ss1IdcNEGf]
  [ss1IdcNEGf] -> Discrete Sample & Hold1/1
  [Intf_sampler] -> Discrete Sample & Hold/2
  [ss1IdcPOSf] -> Discrete Sample & Hold/1
  Add/1 -> [ss2VdcLINK]
  [ss2VdcLINK] -> First-Order Filter/1
  First-Order Filter/1 -> [ss2VdcLINKf]
  [ss2VdcLINKf] -> Discrete Sample & Hold4/1
  [Intf_sampler] -> Discrete Sample & Hold4/2
  [ss1VdcNEG] -> Gain1/1
  [ss1VdcPOS] -> Add1/1
  Gain1/1 -> Add1/2
  Add1/1 -> [ss1VdcLINK]
  [ss1VdcLINK] -> First-Order Filter3/1
  First-Order Filter3/1 -> [ss1VdcLINKf]
  [ss2IdcPOS] -> First-Order Filter4/1
  [ss2IdcNEG] -> First-Order Filter5/1
  First-Order Filter4/1 -> [ss2IdcPOSf]
  First-Order Filter5/1 -> [ss2IdcNEGf]
  [ss2VdcPOS] -> Product/1
  [ss2IdcPOS] -> Product/2
  [ss2VdcNEG] -> Product1/1
  [ss2IdcNEG] -> Product1/2
  Product/1 -> Add2/1
  Product1/1 -> Add2/2
  Add2/1 -> [ss2Pdc]
  [ss2Pdc] -> First-Order Filter6/1
  First-Order Filter6/1 -> [ss2Pdcf]
  [ss1VdcPOS] -> Product2/1
  [ss1IdcPOS] -> Product2/2
  [ss1VdcNEG] -> Product3/1
  [ss1IdcNEG] -> Product3/2
  Product2/1 -> Add3/1
  Product3/1 -> Add3/2
  Add3/1 -> [ss1Pdc]
  [ss1Pdc] -> First-Order Filter7/1
  First-Order Filter7/1 -> [ss1Pdcf]
  [ss1VdcLINKf] -> Bus Creator/3  "ss1VdcLINKf"
  [ss1IdcPOSf] -> Bus Creator/4  "ss1IdcPOSf"
  [ss1IdcNEGf] -> Bus Creator/5  "ss1IdcNEGf"
  [ss1VdcPOSf] -> Bus Creator/1  "ss1VdcPOSf"
  [ss1VdcNEGf] -> Bus Creator/2  "ss1VdcNEGf"
  [ss1Pdcf] -> Bus Creator/6  "ss1Pdcf"
  Bus Creator/1 -> ss1ITMinterface/1
  [ss2VdcLINKf] -> Bus Creator1/3  "ss2VdcLINKf"
  [ss2IdcPOSf] -> Bus Creator1/4  "ss2IdcPOSf"
  [ss2IdcNEGf] -> Bus Creator1/5  "ss2IdcNEGf"
  [ss2VdcPOSf] -> Bus Creator1/1  "ss2VdcPOSf"
  [ss2VdcNEGf] -> Bus Creator1/2  "ss2VdcNEGf"
  [ss2Pdcf] -> Bus Creator1/6  "ss2Pdcf"
  Bus Creator1/1 -> ss2ITMinterface/1
  [ss1VdcPOS] -> First-Order Filter8/1
  First-Order Filter8/1 -> [ss1VdcPOSf]
  [ss1VdcNEG] -> First-Order Filter9/1
  First-Order Filter9/1 -> [ss1VdcNEGf]
  [ss2VdcPOS] -> First-Order Filter10/1
  [ss2VdcNEG] -> First-Order Filter11/1
  First-Order Filter10/1 -> [ss2VdcPOSf]
  First-Order Filter11/1 -> [ss2VdcNEGf]
  connections:
  AC System 2/LConn1 -- B2/LConn1
  AC System 2/LConn2 -- B2/LConn2
  AC System 2/LConn3 -- B2/LConn3
  Station 1 (Rectifier)/LConn1 -- B1/RConn1
  B1/RConn2 -- Station 1 (Rectifier)/LConn2
  Station 1 (Rectifier)/LConn3 -- B1/RConn3
  Station 2 (Inverter)/LConn1 -- B2/RConn1
  Station 2 (Inverter)/LConn2 -- B2/RConn2
  Station 2 (Inverter)/LConn3 -- B2/RConn3
  Ground/LConn1 -- Station 1 (Rectifier)/RConn2
  Ground1/LConn1 -- Station 2 (Inverter)/RConn2
  Ground2/LConn1 -- ss2UdcNEGsrc/LConn1
  ss1IdcPOSmeas/RConn1 -- ss1VdcPOSmeas/LConn1 -- ss2UdcPOSsrc/RConn1
  Ground3/LConn1 -- ss2UdcPOSsrc/LConn1
  ss1IdcNEGmeas/RConn1 -- ss1VdcNEGmeas/LConn1 -- ss2UdcNEGsrc/RConn1
  Ground4/LConn1 -- ss2VdcPOSmeas/LConn2
  Ground5/LConn1 -- ss2IdcPOS/LConn1
  Ground6/LConn1 -- ss2IdcNEG/LConn1
  ss2VdcNEGmeas/LConn2 -- Ground7/LConn1
  ss2IdcNEG/RConn1 -- ss2VdcNEGmeas/LConn1 -- ss2IdcNEGmeas/LConn1
  ss2IdcPOS/RConn1 -- ss2IdcPOSmeas/LConn1 -- ss2VdcPOSmeas/LConn1
  37.5-km cable/RConn1 -- Station 2 (Inverter)/RConn1
  37.5-km  cable/RConn1 -- Station 2 (Inverter)/RConn3
  Station 1 (Rectifier)/RConn1 -- 37.5-km cable1/LConn1
  Station 1 (Rectifier)/RConn3 -- 37.5-km  cable1/LConn1
  ss1VdcPOSmeas/LConn2 -- Ground8/LConn1
  ss1VdcNEGmeas/LConn2 -- Ground9/LConn1
  37.5-km cable1/RConn1 -- ss1IdcPOSmeas/LConn1
  37.5-km  cable1/RConn1 -- ss1IdcNEGmeas/LConn1
  ss2IdcNEGmeas/RConn1 -- 37.5-km  cable/LConn1
  ss2IdcPOSmeas/RConn1 -- 37.5-km cable/LConn1
  AC System 1/RConn3 -- B1/LConn3
  AC System 1/RConn1 -- B1/LConn1
  AC System 1/RConn2 -- B1/LConn2

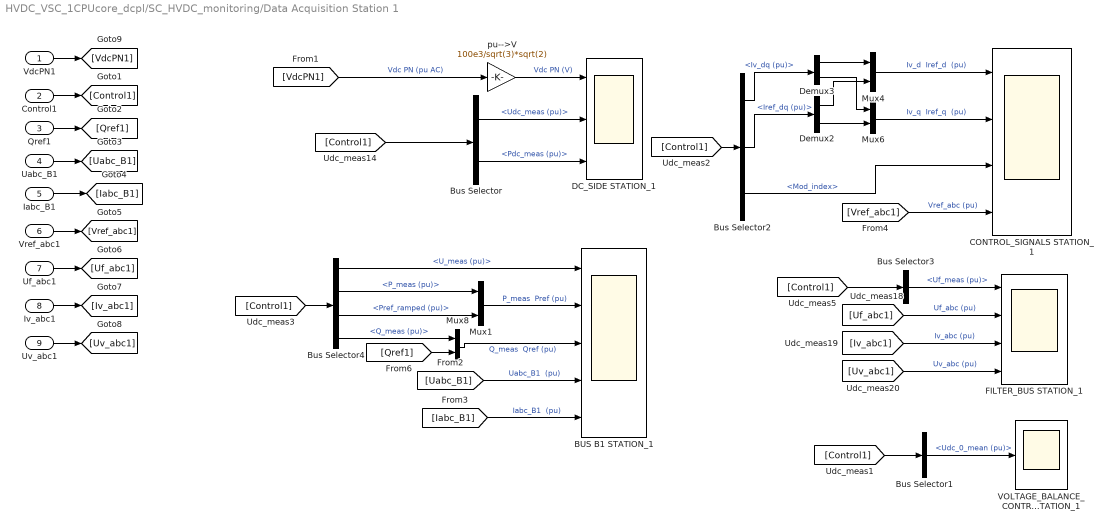
== system HVDC_VSC_1CPUcore_dcpl/SC_HVDC_monitoring/Data Acquisition Station 1 ==
  VdcPN1 : Inport
  Control1 : Inport  Port=2
  Qref1 : Inport  Port=3
  Uabc_B1 : Inport  Port=4
  Iabc_B1 : Inport  Port=5
  Vref_abc1 : Inport  Port=6
  Uf_abc1 : Inport  Port=7
  Iv_abc1 : Inport  Port=8
  Uv_abc1 : Inport  Port=9
  BUS B1 STATION_1 : Scope  NumInputPorts=5
      settings: TimeRange=5  YMin=0.7~-0.3~-0.6~-1.5~-1.5  YMax=1.1~0.3~0.2~1.5~1  SaveName=res_2a  SampleInput=on  SampleTime=Ts_Control
  Bus Selector : BusSelector  OutputSignals=Udc_meas (pu),Pdc_meas (pu)
  Bus Selector1 : BusSelector  OutputSignals=Udc_0_mean (pu)
  Bus Selector2 : BusSelector  OutputSignals=Iv_dq (pu),Iref_dq (pu),Mod_index
  Bus Selector3 : BusSelector  OutputSignals=Uf_meas (pu)
  Bus Selector4 : BusSelector  OutputSignals=U_meas (pu),P_meas (pu),Pref_ramped (pu),Q_meas (pu)
  "CONTROL_SIGNALS STATION_1  " : Scope  NumInputPorts=4
      settings: TimeRange=3  YMin=-0.5~-3~0~-1  YMax=1.5~1~1.5~1  SaveName=ScopeData4  SampleInput=on  SampleTime=Ts_Control
  DC_SIDE STATION_1 : Scope  NumInputPorts=3
      settings: TimeRange=5  YMin=-150000~0.99~-0.497  YMax=150000~1~-0.492  SaveName=ScopeData2  SampleInput=on  SampleTime=Ts_Control
  Demux2 : Demux  Outputs=2
  Demux3 : Demux  Outputs=2
  FILTER_BUS STATION_1 : Scope  NumInputPorts=4
      settings: TimeRange=3  YMin=0~-2~-2~-2  YMax=1.5~2~2~2  SaveName=filter_bus1  Decimation=2  SampleInput=on  SampleTime=Ts_Control
  Mux{1,4,6,8} (4 alike) : Mux  Inputs=2
  VOLTAGE_BALANCE_CONTROL STATION_1 : Scope
      settings: TimeRange=3  YMin=-0.1  YMax=0.04  SaveName=filter_bus  Decimation=2  SampleInput=on  SampleTime=Ts_Control
  pu-->V : Gain  Gain=100e3/sqrt(3)*sqrt(2)
  wires:
  [VdcPN1] -> pu-->V/1  "Vdc PN (pu AC)"
  Demux3/1 -> Mux4/1
  Demux2/1 -> Mux4/2
  Demux3/2 -> Mux6/1
  Demux2/2 -> Mux6/2
  [Uv_abc1] -> FILTER_BUS STATION_1/4  "Uv_abc (pu)"
  [Iv_abc1] -> FILTER_BUS STATION_1/3  "Iv_abc (pu)"
  [Uf_abc1] -> FILTER_BUS STATION_1/2  "Uf_abc (pu)"
  Bus Selector3/1 -> FILTER_BUS STATION_1/1  "<Uf_meas (pu)>"
  Bus Selector/2 -> DC_SIDE STATION_1/3  "<Pdc_meas (pu)>"
  [Control1] -> Bus Selector/1
  Bus Selector/1 -> DC_SIDE STATION_1/2  "<Udc_meas (pu)>"
  Bus Selector4/1 -> BUS B1 STATION_1/1  "<U_meas (pu)>"
  Bus Selector4/2 -> Mux1/1  "<P_meas (pu)>"
  Bus Selector4/3 -> Mux1/2  "<Pref_ramped (pu)>"
  Bus Selector4/4 -> Mux8/1  "<Q_meas (pu)>"
  [Uabc_B1] -> BUS B1 STATION_1/4  "Uabc_B1  (pu)"
  [Iabc_B1] -> BUS B1 STATION_1/5  "Iabc_B1  (pu)"
  Mux1/1 -> BUS B1 STATION_1/2  "P_meas  Pref (pu)"
  Mux8/1 -> BUS B1 STATION_1/3  "Q_meas  Qref (pu)"
  [Control1] -> Bus Selector2/1
  pu-->V/1 -> DC_SIDE STATION_1/1  "Vdc PN (V)"
  Bus Selector2/1 -> Demux3/1  "<Iv_dq (pu)>"
  Bus Selector2/3 -> "CONTROL_SIGNALS STATION_1  "/3  "<Mod_index>"
  [Control1] -> Bus Selector3/1
  Bus Selector2/2 -> Demux2/1  "<Iref_dq (pu)>"
  [Control1] -> Bus Selector1/1
  Bus Selector1/1 -> VOLTAGE_BALANCE_CONTROL STATION_1/1  "<Udc_0_mean (pu)>"
  Mux4/1 -> "CONTROL_SIGNALS STATION_1  "/1  "Iv_d  Iref_d  (pu)"
  Mux6/1 -> "CONTROL_SIGNALS STATION_1  "/2  "Iv_q  Iref_q  (pu)"
  [Vref_abc1] -> "CONTROL_SIGNALS STATION_1  "/4  "Vref_abc (pu)"
  [Qref1] -> Mux8/2
  [Control1] -> Bus Selector4/1
  Control1/1 -> [Control1]
  Qref1/1 -> [Qref1]
  Uabc_B1/1 -> [Uabc_B1]
  Iabc_B1/1 -> [Iabc_B1]
  Vref_abc1/1 -> [Vref_abc1]
  Uf_abc1/1 -> [Uf_abc1]
  Iv_abc1/1 -> [Iv_abc1]
  Uv_abc1/1 -> [Uv_abc1]
  VdcPN1/1 -> [VdcPN1]

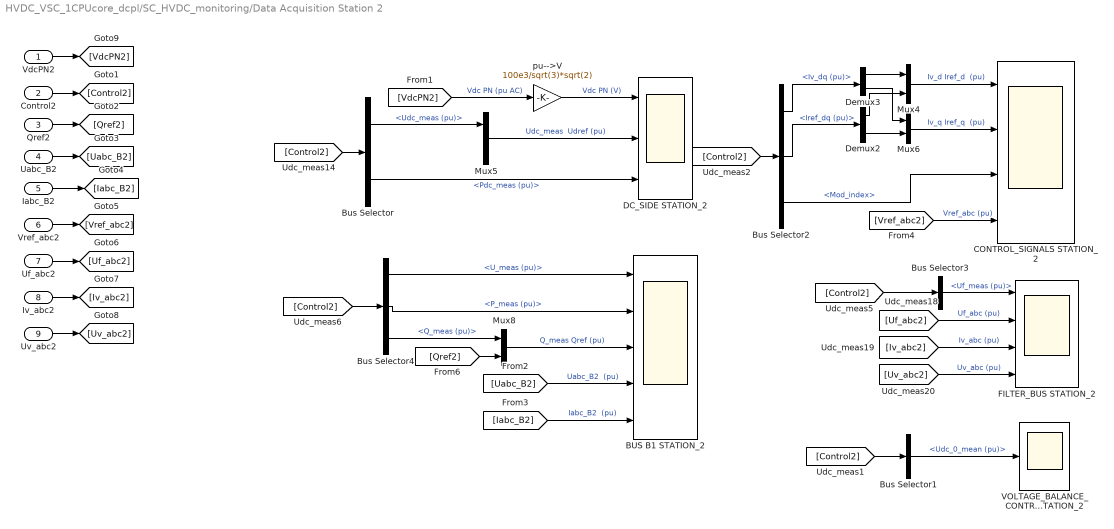
== system HVDC_VSC_1CPUcore_dcpl/SC_HVDC_monitoring/Data Acquisition Station 2 ==
  VdcPN2 : Inport
  Control2 : Inport  Port=2
  Qref2 : Inport  Port=3
  Uabc_B2 : Inport  Port=4
  Iabc_B2 : Inport  Port=5
  Vref_abc2 : Inport  Port=6
  Uf_abc2 : Inport  Port=7
  Iv_abc2 : Inport  Port=8
  Uv_abc2 : Inport  Port=9
  BUS B1 STATION_2 : Scope  NumInputPorts=5
      settings: TimeRange=3  YMin=0.991~0.47~-0.008~-1~-0.5  YMax=0.9925~0.495~0.002~1~0.5  SaveName=res_2b  SampleInput=on  SampleTime=Ts_Control
  Bus Selector : BusSelector  OutputSignals=Udc_meas (pu),Pdc_meas (pu)
  Bus Selector1 : BusSelector  OutputSignals=Udc_0_mean (pu)
  Bus Selector2 : BusSelector  OutputSignals=Iv_dq (pu),Iref_dq (pu),Mod_index
  Bus Selector3 : BusSelector  OutputSignals=Uf_meas (pu)
  Bus Selector4 : BusSelector  OutputSignals=U_meas (pu),P_meas (pu),Q_meas (pu)
  "CONTROL_SIGNALS STATION_2  " : Scope  NumInputPorts=4
      settings: TimeRange=3  YMin=-2~-4~0~-2  YMax=2~2~1.5~2  SaveName=ScopeData4  SampleInput=on  SampleTime=Ts_Control
  DC_SIDE STATION_2 : Scope  NumInputPorts=3
      settings: TimeRange=8  YMin=-148522.64727~-0.14852~-0.05135  YMax=148522.64727~1.33672~0.30732  SaveName=ScopeData2  SampleInput=on  SampleTime=Ts_Control
  Demux2 : Demux  Outputs=2
  Demux3 : Demux  Outputs=2
  FILTER_BUS STATION_2 : Scope  NumInputPorts=4
      settings: TimeRange=3  YMin=0~-2~-4~-4  YMax=1.5~2~4~2  SaveName=filter_bus2  Decimation=2  SampleInput=on  SampleTime=Ts_Control
  Mux{4..6,8} (4 alike) : Mux  Inputs=2
  VOLTAGE_BALANCE_CONTROL STATION_2 : Scope
      settings: TimeRange=3  YMin=-0.1  YMax=0.04  SaveName=filter_bus  Decimation=2  SampleInput=on  SampleTime=Ts_Control
  pu-->V : Gain  Gain=100e3/sqrt(3)*sqrt(2)
  wires:
  [Qref2] -> Mux8/2
  [Vref_abc2] -> "CONTROL_SIGNALS STATION_2  "/4  "Vref_abc (pu)"
  Mux6/1 -> "CONTROL_SIGNALS STATION_2  "/2  "Iv_q Iref_q  (pu)"
  Mux4/1 -> "CONTROL_SIGNALS STATION_2  "/1  "Iv_d Iref_d  (pu)"
  Bus Selector1/1 -> VOLTAGE_BALANCE_CONTROL STATION_2/1  "<Udc_0_mean (pu)>"
  [Control2] -> Bus Selector1/1
  Bus Selector2/2 -> Demux2/1  "<Iref_dq (pu)>"
  [Control2] -> Bus Selector4/1
  [Control2] -> Bus Selector3/1
  Bus Selector2/3 -> "CONTROL_SIGNALS STATION_2  "/3  "<Mod_index>"
  Bus Selector2/1 -> Demux3/1  "<Iv_dq (pu)>"
  pu-->V/1 -> DC_SIDE STATION_2/1  "Vdc PN (V)"
  [Control2] -> Bus Selector2/1
  Mux8/1 -> BUS B1 STATION_2/3  "Q_meas Qref (pu)"
  [Iabc_B2] -> BUS B1 STATION_2/5  "Iabc_B2  (pu)"
  [Uabc_B2] -> BUS B1 STATION_2/4  "Uabc_B2  (pu)"
  Bus Selector4/3 -> Mux8/1  "<Q_meas (pu)>"
  Bus Selector4/1 -> BUS B1 STATION_2/1  "<U_meas (pu)>"
  Bus Selector/1 -> Mux5/1  "<Udc_meas (pu)>"
  [Control2] -> Bus Selector/1
  Bus Selector/2 -> DC_SIDE STATION_2/3  "<Pdc_meas (pu)>"
  Bus Selector3/1 -> FILTER_BUS STATION_2/1  "<Uf_meas (pu)>"
  [Uf_abc2] -> FILTER_BUS STATION_2/2  "Uf_abc (pu)"
  [Iv_abc2] -> FILTER_BUS STATION_2/3  "Iv_abc (pu)"
  [Uv_abc2] -> FILTER_BUS STATION_2/4  "Uv_abc (pu)"
  Demux2/2 -> Mux6/2
  Demux3/2 -> Mux6/1
  Demux2/1 -> Mux4/2
  Demux3/1 -> Mux4/1
  [VdcPN2] -> pu-->V/1  "Vdc PN (pu AC)"
  Mux5/1 -> DC_SIDE STATION_2/2  "Udc_meas  Udref (pu)"
  Bus Selector4/2 -> BUS B1 STATION_2/2  "<P_meas (pu)>"
  Control2/1 -> [Control2]
  Qref2/1 -> [Qref2]
  Uabc_B2/1 -> [Uabc_B2]
  Iabc_B2/1 -> [Iabc_B2]
  Vref_abc2/1 -> [Vref_abc2]
  Uf_abc2/1 -> [Uf_abc2]
  Iv_abc2/1 -> [Iv_abc2]
  Uv_abc2/1 -> [Uv_abc2]
  VdcPN2/1 -> [VdcPN2]

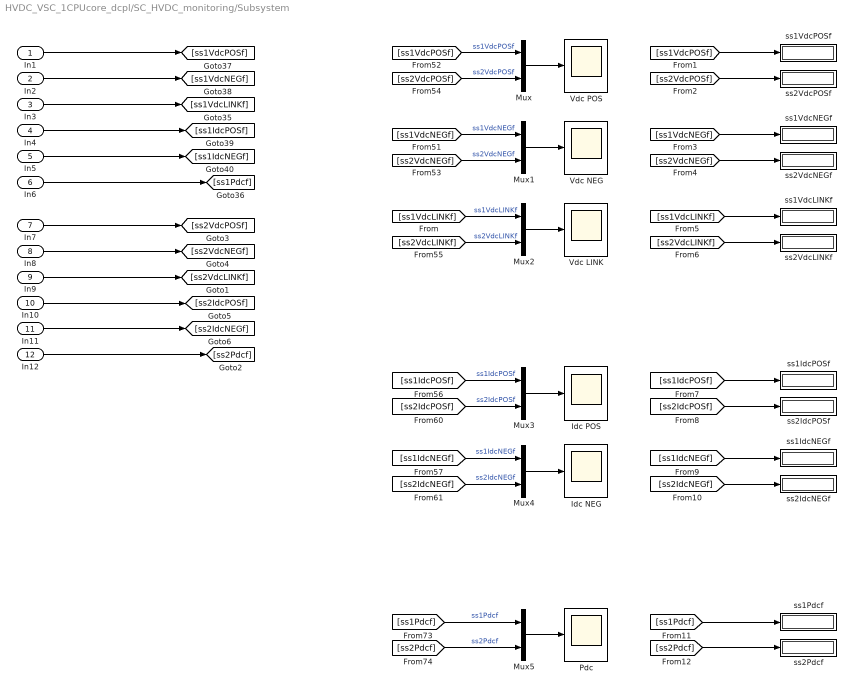
== system HVDC_VSC_1CPUcore_dcpl/SC_HVDC_monitoring/Subsystem ==
  In1 : Inport
  In2 : Inport  Port=2
  In3 : Inport  Port=3
  In4 : Inport  Port=4
  In5 : Inport  Port=5
  In6 : Inport  Port=6
  In7 : Inport  Port=7
  In8 : Inport  Port=8
  In9 : Inport  Port=9
  In10 : Inport  Port=10
  In11 : Inport  Port=11
  In12 : Inport  Port=12
  Idc NEG : Scope
      settings: ShowLegends=on  YMin=-100  YMax=600  SaveName=ScopeData6  ScrollMode=on
  Idc POS : Scope
      settings: ShowLegends=on  YMin=-600  YMax=100  SaveName=ScopeData5  ScrollMode=on
  Mux{,1..5} (6 alike) : Mux  Inputs=2
  Pdc : Scope
      settings: ShowLegends=on  YMin=-4e+07  YMax=1e+08  SaveName=ScopeData7  ScrollMode=on
  Vdc LINK : Scope
      settings: ShowLegends=on  YMin=0  YMax=250000  SaveName=ScopeData3  ScrollMode=on
  Vdc NEG : Scope
      settings: ShowLegends=on  YMin=-120000  YMax=0  ScrollMode=on
  Vdc POS : Scope
      settings: ShowLegends=on  YMin=0  YMax=120000  ScrollMode=on
  ss1IdcNEGf : Display
  ss1IdcPOSf : Display
  ss1Pdcf : Display
  ss1VdcLINKf : Display
  ss1VdcNEGf : Display
  ss1VdcPOSf : Display
  ss2IdcNEGf : Display
  ss2IdcPOSf : Display
  ss2Pdcf : Display
  ss2VdcLINKf : Display
  ss2VdcNEGf : Display
  ss2VdcPOSf : Display
  wires:
  In12/1 -> [ss2Pdcf]
  In1/1 -> [ss1VdcPOSf]
  In3/1 -> [ss1VdcLINKf]
  In2/1 -> [ss1VdcNEGf]
  In4/1 -> [ss1IdcPOSf]
  In6/1 -> [ss1Pdcf]
  In5/1 -> [ss1IdcNEGf]
  In7/1 -> [ss2VdcPOSf]
  In8/1 -> [ss2VdcNEGf]
  In9/1 -> [ss2VdcLINKf]
  In10/1 -> [ss2IdcPOSf]
  In11/1 -> [ss2IdcNEGf]
  [ss1VdcPOSf] -> Mux/1  "ss1VdcPOSf"
  [ss2VdcPOSf] -> Mux/2  "ss2VdcPOSf"
  Mux/1 -> Vdc POS/1
  [ss1VdcPOSf] -> ss1VdcPOSf/1
  [ss2VdcPOSf] -> ss2VdcPOSf/1
  [ss1VdcNEGf] -> Mux1/1  "ss1VdcNEGf"
  [ss2VdcNEGf] -> Mux1/2  "ss2VdcNEGf"
  Mux1/1 -> Vdc NEG/1
  [ss1VdcNEGf] -> ss1VdcNEGf/1
  [ss2VdcNEGf] -> ss2VdcNEGf/1
  [ss1VdcLINKf] -> Mux2/1  "ss1VdcLINKf"
  Mux2/1 -> Vdc LINK/1
  [ss1VdcLINKf] -> ss1VdcLINKf/1
  [ss2VdcLINKf] -> ss2VdcLINKf/1
  [ss2VdcLINKf] -> Mux2/2  "ss2VdcLINKf"
  [ss1IdcPOSf] -> Mux3/1  "ss1IdcPOSf"
  Mux3/1 -> Idc POS/1
  [ss1IdcPOSf] -> ss1IdcPOSf/1
  [ss2IdcPOSf] -> ss2IdcPOSf/1
  [ss2IdcPOSf] -> Mux3/2  "ss2IdcPOSf"
  [ss1IdcNEGf] -> Mux4/1  "ss1IdcNEGf"
  Mux4/1 -> Idc NEG/1
  [ss1IdcNEGf] -> ss1IdcNEGf/1
  [ss2IdcNEGf] -> ss2IdcNEGf/1
  [ss2IdcNEGf] -> Mux4/2  "ss2IdcNEGf"
  Mux5/1 -> Pdc/1
  [ss1Pdcf] -> Mux5/1  "ss1Pdcf"
  [ss2Pdcf] -> Mux5/2  "ss2Pdcf"
  [ss1Pdcf] -> ss1Pdcf/1
  [ss2Pdcf] -> ss2Pdcf/1
